simulink model "ex_1"  (R2018a)
settings: Solver=VariableStepAuto  StartTime=0.0  StopTime=10.0  RelTol=1e-3
settings Model: Creator=80741  LastModifiedBy=80741

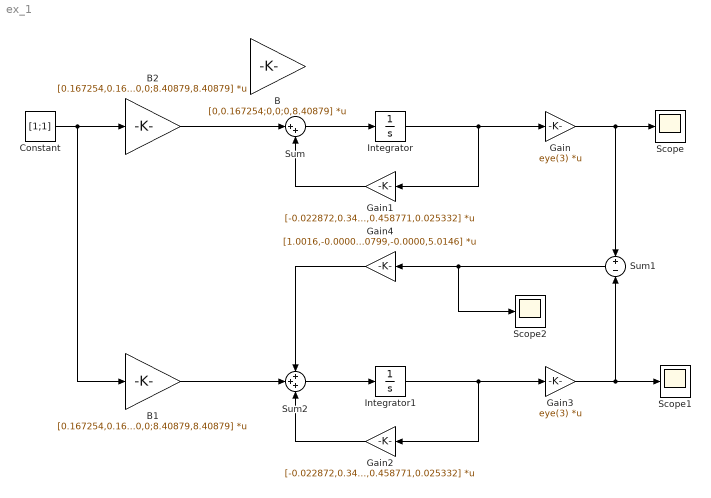
== system ex_1 ==
  B : Gain  Gain=[0,0.167254;0,0;0,8.40879]  Multiplication=Matrix(K*u) (u vector)
  B1 : Gain  Gain=[0.167254,0.167254;0,0;8.40879,8.40879]  Multiplication=Matrix(K*u) (u vector)
  B2 : Gain  Gain=[0.167254,0.167254;0,0;8.40879,8.40879]  Multiplication=Matrix(K*u) (u vector)
  Constant : Constant  Value=[1;1]
  Gain : Gain  Gain=eye(3)  Multiplication=Matrix(K*u) (u vector)
  Gain1 : Gain  Gain=[-0.022872,0.34878,0;0,0,1;-0.458771,0.458771,0.025332]  Multiplication=Matrix(K*u) (u vector)
  Gain2 : Gain  Gain=[-0.022872,0.34878,0;0,0,1;-0.458771,0.458771,0.025332]  Multiplication=Matrix(K*u) (u vector)
  Gain3 : Gain  Gain=eye(3)  Multiplication=Matrix(K*u) (u vector)
  Gain4 : Gain  Gain=[1.0016,-0.0000,0.0791; 0.0199,1.0000,0.9996; 0.0799,-0.0000,5.0146]  Multiplication=Matrix(K*u) (u vector)
  Integrator : Integrator
  Integrator1 : Integrator
  Scope : Scope
  Scope1 : Scope
  Scope2 : Scope
  Sum : Sum  Inputs=|++
  Sum1 : Sum  Inputs=+-
  Sum2 : Sum  Inputs=+++
  wires:
  B2/1 -> Sum/1
  Sum/1 -> Integrator/1
  Integrator/1 -> Gain1/1, Gain/1
  Gain/1 -> Sum1/1, Scope/1
  Gain1/1 -> Sum/2
  Constant/1 -> B2/1, B1/1
  Integrator1/1 -> Gain3/1, Gain2/1
  Gain3/1 -> Scope1/1, Sum1/2
  Sum1/1 -> Scope2/1, Gain4/1
  Gain4/1 -> Sum2/1
  Gain2/1 -> Sum2/3
  B1/1 -> Sum2/2
  Sum2/1 -> Integrator1/1
